simulink model "untitled"  (R2018b)
settings: Solver=FixedStepDiscrete  StartTime=0.0  StopTime=10.0  RelTol=1e-3
settings Model: Creator=karim  LastModifiedBy=karim

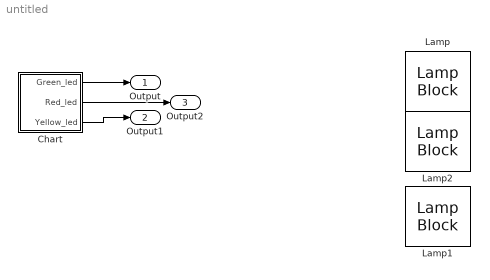
== system untitled ==
  Chart : Stateflow chart  TreatAsAtomicUnit=on
  Lamp : LampBlock  WebBlockId=11
  Lamp1 : LampBlock  WebBlockId=12
  Lamp2 : LampBlock  WebBlockId=13
  Output : Outport
  Output1 : Outport  Port=2
  Output2 : Outport  Port=3
  wires:
  Chart/3(Yellow_led) -> Output1/1
  Chart/1(Green_led) -> Output/1
  Chart/2(Red_led) -> Output2/1

== stateflow chart untitled/Chart ==
  state Yellow
    en:
    Yellow_led=1;
    Red_led=0;
    Green_led=0;
    du:
    Yellow_led=1;
    ex:
    Yellow_led=0;
  state Red
    en:
    Red_led=1;
    Yellow_led=0;
    Green_led=0;
    du:
    Red_led=1;
    ex:
    Red_led=0;
  state Green
    en:
    Green_led=1;
    Red_led=0;
    Yellow_led=0;
    du:
    Green_led=1;
    ex:
    Green_led=0;
  (default) -> Red
  Red -> Yellow : [after(3,sec)]
  Green -> Red : [after(3,sec)]
  Yellow -> Green : [after(3,sec)]
  data: Green_led output double; Red_led output double; Yellow_led output double
